simulink model "furuta_pendulum_c"  (R2016a)
settings: Solver=VariableStepAuto  StartTime=0.0  StopTime=10.0  RelTol=1e-3
undefined symbols (not defined in the file): alpha, beta, delta, dq0, gamma, la, lp, q0
settings Model: Creator=mgreiff  LastModifiedBy=mgreiff
settings DataIOCC: LimitDataPoints=on
settings DebuggingCC: AllowSymbolicDim=off
settings ModelReferenceCC: PropagateSignalLabelsOutOfModel=off
settings GRTTargetCC: GeneratePreprocessorConditionals=Use local settings

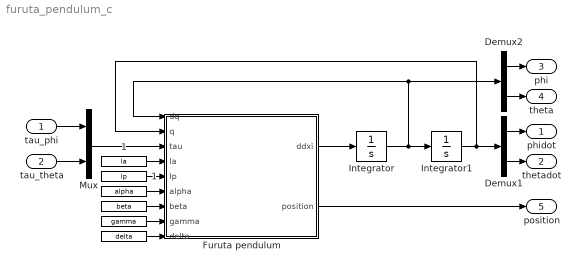
== system furuta_pendulum_c ==
  tau_phi : Inport  PortDimensions=1
  tau_theta : Inport  Port=2  PortDimensions=1
  " " : Constant  Value=alpha
  "  " : Constant  Value=beta
  "   " : Constant  Value=gamma
  "    " : Constant  Value=delta
  "  1" : Constant  Value=lp
  " 1" : Constant  Value=la
  Demux1 : Demux  Outputs=2
  Demux2 : Demux  Outputs=2
  Furuta pendulum : MATLAB Function  TreatAsAtomicUnit=on
  Integrator : Integrator  InitialCondition=dq0
  Integrator1 : Integrator  InitialCondition=q0
  Mux : Mux  Inputs=2
  "phidot " : Outport  PortDimensions=1
  thetadot : Outport  Port=2  PortDimensions=1
  phi : Outport  Port=3  PortDimensions=1
  theta : Outport  Port=4  PortDimensions=1
  "position " : Outport  Port=5  PortDimensions=3
  wires:
  Furuta pendulum/1(ddxi) -> Integrator/1
  Integrator/1 -> Demux2/1, Furuta pendulum/1(dq), Integrator1/1
  Integrator1/1 -> Furuta pendulum/2(q), Demux1/1
  tau_phi/1 -> Mux/1
  tau_theta/1 -> Mux/2
  Mux/1 -> Furuta pendulum/3(tau)
  " "/1 -> Furuta pendulum/6(alpha)
  "  "/1 -> Furuta pendulum/7(beta)
  "   "/1 -> Furuta pendulum/8(gamma)
  "    "/1 -> Furuta pendulum/9(delta)
  Demux1/2 -> thetadot/1
  Demux1/1 -> "phidot "/1
  Demux2/2 -> theta/1
  Demux2/1 -> phi/1
  " 1"/1 -> Furuta pendulum/4(la)
  "  1"/1 -> Furuta pendulum/5(lp)
  Furuta pendulum/2(position) -> "position "/1

== matlab function furuta_pendulum_c/Furuta pendulum ==
  data: dq input; q input; tau input; la input; lp input; ddxi output; alpha input; beta input; gamma input; delta input; position output
function [ddxi, position]= fcn(dq, q, tau, la, lp, alpha, beta, gamma, delta)
%#codegen
phi    = q(1);
theta  = q(2);
dphi   = dq(1);
dtheta = dq(2);

cp = cos(phi);
sp = sin(phi);
ct = cos(theta);
st = sin(theta);

D = [alpha + beta*(st.^2), gamma * ct;
     gamma * ct          , beta     ];
C = [ beta * ct * st * dtheta, beta * ct * st * dphi - gamma * st * dtheta;
     -beta * ct * st * dphi  , 0                                         ];
g = [0; -delta * st];

ddxi = D \ (tau - C * [dphi; dtheta] - g);

% Compute position in globalcoordinates for debugging
x = la * cp - lp * sp * st;
y = la * sp + lp * cp * st;
z = lp * ct;
position = [x;y;z];
end
